simulink model "Motors_Simulink_Gripper"  (R2019b)
settings: Solver=VariableStepAuto  StartTime=0.0  StopTime=2  FixedStep=0.0001  RelTol=1e-3
values from neighbouring files (symbols this model uses):
  WKb = Kb(2)    [Motors_gripper_Code.m]
  WKm = Km(2)    [Motors_gripper_Code.m]
  WL = L(2)    [Motors_gripper_Code.m]
undefined symbols (not defined in the file or in its folder): GR
libraries: cstblocks x1
settings Model: Creator=harsh  LastModifiedBy=debby

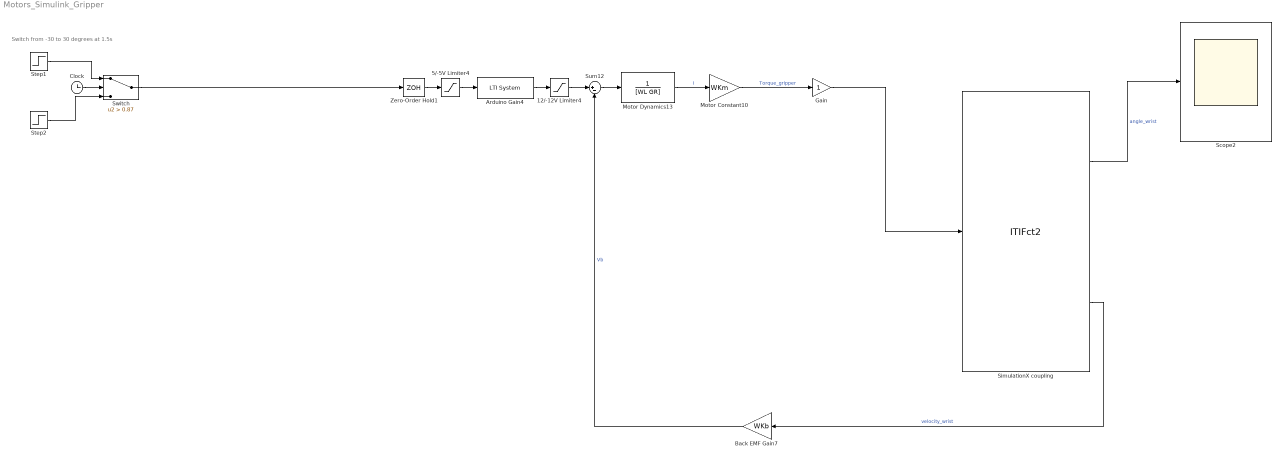
== system Motors_Simulink_Gripper ==
  note: Switch from -30 to 30 degrees at 1.5s
  12/-12V Limiter4 : Saturate  UpperLimit=12  LowerLimit=-12
  5/-5V Limiter4 : Saturate  UpperLimit=5  LowerLimit=-5
  Arduino Gain4 : cstblocks/LTI System  sys=GOPAMP  IC=[]
  Back EMF Gain7 : Gain  Gain=WKb
  Clock : Clock
  Gain : Gain
  Motor Constant10 : Gain  Gain=WKm
  Motor Dynamics13 : TransferFcn  Denominator=[WL GR]
  Scope2 : Scope
  SimulationX coupling : S-Function  FunctionName=ITIFct2  Parameters=ip, port, ts, nIn, nOut  SFunctionDeploymentMode=off  EnableBusSupport=off  mask{ip='localhost', port=1025, ts=0.001, nIn=1, nOut=2}
      mask prompts: ip "Address: ip"; port "Port Number: port [-]"; ts "Communication Step Size: ts [s]"; nIn "Input Vector Dimension (to SimulationX): nIn [-]"; nOut "Output Vector Dimension (from SimulationX): nOut [-]"
      mask help: Coupling Element
  Step1 : Step  Time=0  After=1.5  SampleTime=0
  Step2 : Step  Time=0  After=-1  SampleTime=0
  Sum12 : Sum  Inputs=|+-
  Switch : Switch  Criteria=u2 > Threshold  Threshold=0.87
  Zero-Order Hold1 : ZeroOrderHold  SampleTime=0.0001
  wires:
  5/-5V Limiter4/1 -> Arduino Gain4/1
  Arduino Gain4/1 -> 12/-12V Limiter4/1
  Back EMF Gain7/1 -> Sum12/2  "Vb"
  Sum12/1 -> Motor Dynamics13/1
  12/-12V Limiter4/1 -> Sum12/1
  Motor Dynamics13/1 -> Motor Constant10/1  "I"
  Motor Constant10/1 -> Gain/1  "Torque_gripper"
  Zero-Order Hold1/1 -> 5/-5V Limiter4/1
  SimulationX coupling/1 -> Scope2/1  "angle_wrist"
  SimulationX coupling/2 -> Back EMF Gain7/1  "velocity_wrist"
  Gain/1 -> SimulationX coupling/1
  Clock/1 -> Switch/2
  Step1/1 -> Switch/1
  Step2/1 -> Switch/3
  Switch/1 -> Zero-Order Hold1/1
